simulink library "SUB_ECU_L4_MABX_HW_Interface_PTC_166"  (R2018a)
settings: Solver=VariableStepAuto  StartTime=0.0  StopTime=10.0  RelTol=1e-3
PostLoadFcn:
  | , if any(exist('dsrtsu_mdlpostloadfcn', 'file') == [2, 3, 6]), try dsrtsu_mdlpostloadfcn('Execute', bdroot); catch fprintf('Error in PostLoadFcn (dsrtsu_mdlpostloadfcn) for model "%s":\n %s\n', bdroot, lasterr); end, end,
undefined symbols (not defined in the file or in its folder): CANR_PROPB_REAX_3_13_CHANNEL_APV, CANR_PROPB_REAX_4_13_CHANNEL_APV, CANR_PROPB_XPR_1_50_CHANNEL_APV, ENUM_CAN_RX_T, ENUM_CAN_TX_T, ENUM_REAX_OPERATION_MODE_T, ENUM_SIGNAL_HEALTH_T, ENUM_XBR_CONTROL_MODE_T, ENUM_XBR_EBI_MODE_T, ENUM_XBR_PASS_THROUGH_ACTIVE_T, ENUM_XBR_PRIORITY_T, ENUM_XPR_INHIBIT_PARK_MANUAL_T, ENUM_XPR_INHIBIT_UNPARK_MANUAL_T, ENUM_XPR_PARK_MANUAL_T, ENUM_XPR_UNPARK_MANUAL_T, PROPB_REAX_1_E4_DES_POS_SIG_SRC_APV, PROPB_REAX_1_E4_DESIRED_OPMODE_APV, PROPB_REAX_1_E4_DESIRED_POSITION_APV, ptc_matlab_lib
libraries: PTC_MBDS_LIB x163, rtican x79, simulink x41, EmE_MBD_Blockset x35, rti1401lib_dio_type4 x8, simulink_need_slupdate x7, $bdroot x5, rti1401lib_adc_type4 x3, rtitasklib x1
(part 25 of 25)

== system SUB_ECU_L4_MABX_HW_Interface_PTC_166/CAN_Out_PTC_166/CAN_TX_5000ms/CAN_TX_RQST_13_E4/TX_CAN5 ==
  Enable : Inport
  RawData : Inport  Port=2
  OperatorEnable : Inport  Port=3
  AND : PTC_MBDS_LIB/MBDS Standard Library/Basic Operations/Logic and Bit Operations/AND  BitwiseMode=off  Inputs=2  UseBitMask=off  BitMask='A7'  OutDataTypeStr=Inherit: Inherit via back propagation  PTC_MBDS_BlockVersion=5.41  PTC_BlockType=PTC_MBDS_AND
      settings: SourceProductName=PACCAR Technical Center MBDS Library
  Data Type Conversion : DataTypeConversion
  Data Type Conversion1 : DataTypeConversion
  Data Type Conversion2 : DataTypeConversion
  Demux : Demux  Outputs=3
  RQST_13_E4 : rtican/RTICAN Transmit (TX)   Reserved1=[]  Reserved2=[]  Reserved3=[]  Reserved4=[]  SfcnMessage=[]  Msg_Struct=[]  BoardTypeNo=[]  BoardNo=[]  ChannelNo=[]  Parameters=[]  DialogFcn=[]  UnitName=[]  Revision=[]  UnitValues=[]  DSProperties=struct('RTI',struct('Version',uint32(5),'BlockType',struct('isSLSource',uint8(1),'isSLSink',uint8(1),'isHWSource',uint8(0),'isHWSink',uint8(0),'isSetup',uint8(0),'isInline',uint8(1),'isNonInline',uint8(0),'isInterrupt',uint8(0),'isChannelwise',uint8(0)),'IOBoardType','RTICAN','UnitType','MESSAGE','Identifier','TX','DialogType','MSVC','BlockSet','RTICAN','SlaveProcessor','CAN'))  RTIBlockInterface=struct('InputPortsWidth',int32([1 1 1]),'InputPortsActive',[1 1 1],'InputPortsName',{{'byte1','byte2','byte3'}},'InputPortsDataType',{{'SS_DOUBLE','SS_DOUBLE','SS_DOUBLE'}},'OutputPortsWidth',int32([1 1 1 1]),'OutputPortsActive',[1 1 1 1],'OutputPortsName',{{['TX status'],['TX time'],['TX delta time'],['TX delay time']}},'DialogFcn','rtican_message_interface_gui','BlockDisplay',{{'','center'}},'IconTransparency','on','InitLevel',3,'BlockName',struct('Token',{{'RQST_13_E4'}}),'SampleTime',{{-1}},'TriggerPort',{{'none'}},'EnablePort',{{'yes'}})  RTIBlockParameters=struct('BoardTypeNo',{{1,'OFF',[]}},'BoardNo',{{3,'ON',[1 16]}},'ChannelNo',{{1,'ON',[1 2]}},'Parameters',{{struct('DataFileSupport',struct('DataFileSelectedMaster',1,'DataFileSelectedLocal',0,'DataFileName','c:\data\svn\truck1571\dbc\mabx_can4_chrisbaltonallstandard.dbc|c:\data\svn\truck1571\dbc\mabx_can4.dbc|','DataFileDate',{{{['11-Nov-2016 14:30:51']}}},'SelectedFile',['<no file selected>']),'Options',struct('StatusSelected',1,'TimeSelected',1,'DeltaTimeSelected',1,'DelayTimeSelected',1,'DelayTimeTXCommandSelected',0,'EncodeSetUnusedBitsToOne',0,'EnableMsgLoopback',0,'TriggerPort',struct('Selected',0,'TriggerType',0),'EnablePortSelected',1,'SignalOnPortnameSelected',1,'UserCoding',struct('Selected',0,'InterfaceFile','UserEncodingFile','FcnName','UserEncodeFcn','InportSelected',0,'InportWidth',1,'OutportSelected',0,'OutportWidth',1),'TerminationMsg',struct('Selected',0,'Byte0_7','0'),'InitialMsg',struct('Selected',0,'Byte0_7','0')),'Message',struct('MsgOnBlocknameSelected',1,'MsgName','RQST_13_E4','MsgIdFormat',1,'MsgId',417993700,'MsgLength',8,'NumSignals',3,'SampleTime',-1,'StartTime',struct('Selected',0,'Value',0),'AutoRepeatTime',struct('Selected',0,'Value',0.1),'Timeout',struct('Selected',0,'Value',0.1),'DelayTime',struct('Selected',0,'Value',0.1),'Signal',struct('SgnName',{'byte1','byte2','byte3'},'SgnStartBit',{0,8,16},'SgnLength',{8,8,8},'SgnType',{0,0,0},'ModeValue',{-1,-1,-1},'DataType',{0,0,0},'ByteLayout',{0,0,0},'Factor',{1,1,1},'Offset',{0,0,0},'SgnComment',{{''},{''},{''}},'SgnUnit',{'','',''},'Min',{0,0,0},'Max',{0,0,0},'SLDataType',{'SS_DOUBLE','SS_DOUBLE','SS_DOUBLE'}),'MsgIdNumFormat',1,'MsgComment',{{['Request message 1']}}),'Version',1.2,'general',struct('isFromLib',0)),'OFF',[]}},'GroupId',{{struct('Group',{{'RTICAN'}},'No',5,'Behavior',{{'NAMECHANGE'}},'BlockType',{{'SINK'}},'NameChangeFlag',0),'OFF',[]}},'SFcnRTICANMessage',{{struct('MsgType','TX','SFcnPortType','Scalar','MsgName','RQST_13_E4','MsgIdFormat','XTD','MsgId',417993700,'MsgLength',8,'NumSignals',3,'SampleTime',-1,'StartTime',struct('Selected','no','Value',0),'AutoRepeatTime',struct('Selected','no','Value',0.1),'Timeout',struct('Selected','no','Value',0.1),'Signal',struct('SgnName',{'byte1','byte2','byte3'},'SgnStartBit',{0,8,16},'SgnLength',{8,8,8},'SgnType',{'standard','standard','standard'},'ModeValue',{-1,-1,-1},'DataType',{['unsigned int'],['unsigned int'],['unsigned int']},'ByteLayout',{['little endian'],['little endian'],['little endian']},'Factor',{1,1,1},'Offset',{0,0,0},'SLDataType',{'SS_DOUBLE','SS_DOUBLE','SS_DOUBLE'}),'StatusSelected','yes','TimeSelected','yes','DeltaTimeSelected','yes','DelayTimeSelected','yes','DelayTimeTXCommandSelected','no','EncodeSetUnusedBitsToOne','no','EnableMsgLoopback','no','TriggerPort',struct('Selected','no','TriggerType',0),'EnablePortSelected','yes','UserCoding',struct('Selected','no','InterfaceFile','UserEncodingFile','FcnName','UserEncodeFcn','InportSelected','no','InportWidth',1,'OutportSelected','no','OutportWidth',1),'TerminationMsg',struct('Selected','no','Byte0','0x00','Byte1','0x00','Byte2','0x00','Byte3','0x00','Byte4','0x00','Byte5','0x00','Byte6','0x00','Byte7','0x00'),'InitialMsg',struct('Selected','no','Byte0','0x00','Byte1','0x00','Byte2','0x00','Byte3','0x00','Byte4','0x00','Byte5','0x00','Byte6','0x00','Byte7','0x00'),'BoardType','DS1','BoardNo',3,'ControllerNo',1),'OFF',[]}},'TLCFileName',{{'rtican_tx_message','OFF',[]}})  RTISFcnParameters=struct('SFcnRTICANMessage','struct','TLCFileName','char')  RTIBlockParaDefault=struct('BoardTypeNo',4302,'BoardNo',1,'ChannelNo',1,'Parameters',struct('DataFileSupport',struct('DataFileSelectedMaster',0,'DataFileSelectedLocal',0,'DataFileName','','DataFileDate','','SelectedFile',['<no file selected>']),'Options',struct('StatusSelected',1,'TimeSelected',1,'DeltaTimeSelected',1,'DelayTimeSelected',1,'DelayTimeTXCommandSelected',0,'EncodeSetUnusedBitsToOne',0,'EnableMsgLoopback',0,'TriggerPort',struct('Selected',0,'TriggerType','rising'),'EnablePortSelected',0,'SignalOnPortnameSelected',1,'UserCoding',struct('Selected',0,'InterfaceFile','UserEncodingFile','FcnName','UserEncodeFcn','InportSelected',0,'InportWidth',1,'OutportSelected',0,'OutportWidth',1),'TerminationMsg',struct('Selected',0,'Byte0_7','0'),'InitialMsg',struct('Selected',0,'Byte0_7','0')),'Message',struct('MsgOnBlocknameSelected',0,'MsgName',['TX Message'],'MsgIdFormat',0,'MsgId',100,'MsgLength',8,'NumSignals',1,'SampleTime',-1,'StartTime',struct('Selected',0,'Value',0),'AutoRepeatTime',struct('Selected',0,'Value',0.1),'Timeout',struct('Selected',0,'Value',0.1),'DelayTime',struct('Selected',0,'Value',0.1),'Signal',struct('SgnName',['TX signal'],'SgnStartBit',0,'SgnLength',8,'SgnType',0,'ModeValue',-1,'DataType',0,'SLDataType','SS_DOUBLE','ByteLayout',0,'Factor',1,'Offset',0,'Min',0,'Max',255,'SgnComment',{{}},'SgnUnit',''),'MsgIdNumFormat',0,'MsgComment',{{''}}),'Version',1.2,'general',struct('isFromLib',1)),'GroupId',struct('Group',{{'RTICAN'}},'No',1,'Behavior',{{'NAMECHANGE'}},'BlockType',{{'SINK'}},'NameChangeFlag',0),'SFcnRTICANMessage',struct('MsgType','TX','MsgName',['TX Message'],'MsgIdFormat','STD','MsgId',100,'MsgLength',2,'NumSignals',1,'SampleTime',-1,'StartTime',struct('Selected','no','Value',0),'AutoRepeatTime',struct('Selected','no','Value',0.1),'Timeout',struct('Selected','no','Value',0.1),'DelayTime',struct('Selected','no','Value',0.1),'Signal',struct('SgnName',['TX signal'],'SgnStartBit',0,'SgnLength',8,'SgnType','standard','ModeValue',-1,'DataType',['unsigned int'],'ByteLayout',['little endian'],'SLDataType','SS_DOUBLE','Factor',1,'Offset',0),'StatusSelected','yes','TimeSelected','yes','DeltaTimeSelected','yes','DelayTimeSelected','yes','EnablePortSelected','no','EnableMsgLoopback','no','DelayTimeTXCommandSelected','no','EncodeSetUnusedBitsToOne','no','UserCoding',struct('Selected','no','InterfaceFile','UserDecodingFile','FcnName','UserDecodeFcn','InportSelected','no','InportWidth',1,'OutportSelected','no','OutportWidth',1),'TerminationMsg',struct('Selected','no','Byte0','0x00','Byte1','0x00','Byte2','0x00','Byte3','0x00','Byte4','0x00','Byte5','0x00','Byte6','0x00','Byte7','0x00'),'InitialMsg',struct('Selected','no','Byte0','0x00','Byte1','0x00','Byte2','0x00','Byte3','0x00','Byte4','0x00','Byte5','0x00','Byte6','0x00','Byte7','0x00'),'TriggerPort',struct('Selected','no','TriggerType','rising'),'BoardType','DS4302','BoardNo',1,'ControllerNo',1,'SFcnPortType','Scalar'),'TLCFileName','rtican_tx_message')
      settings: AttributesFormatString=Group Id: RTICAN5\n  SourceProductName=dSPACE RTI CAN Blockset
  Terminator{,1..3} (4 alike) : Terminator
      settings: InitFcn=|
      | try
      |    MBDS_BlockCallback('Update', gcb);
      | end
  wires:
  Data Type Conversion2/1 -> RQST_13_E4/3
  Data Type Conversion1/1 -> RQST_13_E4/2
  Data Type Conversion/1 -> RQST_13_E4/1
  AND/1 -> RQST_13_E4/Enable
  OperatorEnable/1 -> AND/2
  Demux/3 -> Data Type Conversion2/1
  Demux/2 -> Data Type Conversion1/1
  Demux/1 -> Data Type Conversion/1
  RQST_13_E4/1 -> Terminator/1
  RQST_13_E4/3 -> Terminator2/1
  Enable/1 -> AND/1
  RQST_13_E4/4 -> Terminator3/1
  RQST_13_E4/2 -> Terminator1/1
  RawData/1 -> Demux/1

== system SUB_ECU_L4_MABX_HW_Interface_PTC_166/CAN_Out_PTC_166/CAN_TX_VariableRate/CAN_TX_Std_SystemTime_01/TX_CAN6 ==
  Enable : Inport
  Data : Inport  Port=2
  AND : PTC_MBDS_LIB/MBDS Standard Library/Basic Operations/Logic and Bit Operations/AND  BitwiseMode=off  Inputs=2  UseBitMask=off  BitMask='A7'  OutDataTypeStr=Inherit: Inherit via back propagation  PTC_MBDS_BlockVersion=5.41  PTC_BlockType=PTC_MBDS_AND
      settings: SourceProductName=PACCAR Technical Center MBDS Library
  Bus Selector : BusSelector  OutputSignals=INPUTS.CAN.SystemTime.RX_status,INPUTS.CAN.SystemTime.SID,INPUTS.CAN.SystemTime.Source,INPUTS.CAN.SystemTime.Date,INPUTS.CAN.SystemTime.Time
  Constant : Constant  Value=0
  Constant1 : Constant
  Std_SystemTime_01 : rtican/RTICAN Transmit (TX)   Reserved1=[]  Reserved2=[]  Reserved3=[]  Reserved4=[]  SfcnMessage=[]  Msg_Struct=[]  BoardTypeNo=[]  BoardNo=[]  ChannelNo=[]  Parameters=[]  DialogFcn=[]  UnitName=[]  Revision=[]  UnitValues=[]  DSProperties=struct('RTI',struct('Version',uint32(5),'BlockType',struct('isSLSource',uint8(1),'isSLSink',uint8(1),'isHWSource',uint8(0),'isHWSink',uint8(0),'isSetup',uint8(0),'isInline',uint8(1),'isNonInline',uint8(0),'isInterrupt',uint8(0),'isChannelwise',uint8(0)),'IOBoardType','RTICAN','UnitType','MESSAGE','Identifier','TX','DialogType','MSVC','BlockSet','RTICAN','SlaveProcessor','CAN'))  RTIBlockInterface=struct('InputPortsWidth',int32([1 1 1 1 1 1]),'InputPortsActive',[1 1 1 1 1 1],'InputPortsName',{{'SID','Source','Date','Time',['Delay TX command'],'Loop-back'}},'InputPortsDataType',{{'SS_DOUBLE','SS_DOUBLE','SS_DOUBLE','SS_DOUBLE','SS_DOUBLE','SS_DOUBLE'}},'OutputPortsWidth',int32([1 1 1 1]),'OutputPortsActive',[1 1 1 1],'OutputPortsName',{{['TX status'],['TX time'],['TX delta time'],['TX delay time']}},'DialogFcn','rtican_message_interface_gui','BlockDisplay',{{'','center'}},'IconTransparency','on','InitLevel',3,'BlockName',struct('Token',{{'Std_SystemTime_01'}}),'SampleTime',{{-1}},'TriggerPort',{{'none'}},'EnablePort',{{'yes'}})  RTIBlockParameters="struct('BoardTypeNo',{{1,'OFF',[]}},'BoardNo',{{3,'ON',[1 16]}},'ChannelNo',{{2,'ON',[1 2]}},'Parameters',{{struct('DataFileSupport',struct('DataFileSelectedMaster',1,'DataFileSelectedLocal',1,'DataFileName','c:\\localdata\\chris\\advanced_tech\\adas\\level4_rcp\\truck1571\\dbc\\mabx_can6.dbc|c:\\localdata\\chris\\advanced_tech\\adas\\level4_rcp\\candb\\mabx_can4_chrisbalton.dbc|','DataFileDate',['15-Feb-2018 08:21:11'],'SelectedFile','dbc\\mabx_can6_beta4.dbc','InterfaceFcn','rtican_dbc_file_parser'),'Options',struct('StatusSelected',1,'TimeSelected',1,'DeltaTimeSelected',1,'DelayTimeSelected',1,'DelayTimeTXCommandSelected',1,'EncodeSetUnusedBitsToOne',0,'EnableMsgLoopback',1,'TriggerPort',struct('Selected',0,'TriggerType',0),'EnablePortSelected',1,'SignalOnPortnameSelected',1,'UserCoding',struct('Selected',0,'InterfaceFile','UserEncodingFile','FcnName','UserEncodeFcn','InportSelected',0,'InportWidth',1,'OutportSelected',0,'OutportWidth',1),'TerminationMsg',struct('Selected',0,'Byte0_7','0'),'InitialMsg',struct('Selected',0,'Byte0_7','0')),'Message',struct('MsgOnBlocknameSelected',1,'MsgName','Std_SystemTime_01','MsgIdFormat',0,'MsgId',5,'MsgLength',8,'NumSignals',4,'SampleTime',-1,'StartTime',struct('Selected',0,'Value',0),'AutoRepeatTime',struct('Selected',0,'Value',0.1),'Timeout',struct('Selected',0,'Value',0.1),'DelayTime',struct('Selected',0,'Value',0.1),'Signal',struct('SgnName',{'SID','Source','Date','Time'},'SgnStartBit',{0,8,16,32},'SgnLength',{8,4,16,32},'ByteLayout',{0,0,0,0},'Factor',{1,1,1,0.0001},'Offset',{0,0,0,0},'SgnComment',{['An upward counting number used to tie related information together between different PGNs.For example,SID would be used to tie together COG,SOG and RAIM values to a given Pos.255=no valid Pos fix to tie it to.Range 0 to 250 for valid Pos fixes.'],['0x0 = GPS, ' char(10) '0x1 =GLONASS, ' char(10) '0x2 = WWV or equivalent Radio Station Time Sync, ' char(10) '0x3 = Local Cesium clock, ' char(10) '0x4 = Local Rubidium clock, ' char(10) '0x5 = Local Crystal clock, ' char(10) '0x6 - 0xE = reserved, ' char(10) '0xF = Null'],['Days since January 1, 1970,   Date is relative to UTC Time.'],['24 hour clock, 0 =  midnight,  time is in UTC']},'SgnUnit',{'','','day','sec'},'Min',{0,0,0,0},'Max',{252,15,65532,86401},'SgnType',{0,0,0,0},'SLDataType',{'SS_DOUBLE','SS_DOUBLE','SS_DOUBLE','SS_DOUBLE'},'DataType',{0,0,0,0},'ModeValue',{-1,-1,-1,-1}),'MsgIdNumFormat',0,'MsgComment',{{['The purpose of this PGN is twofold:' char(10) '' char(10) '- To provide a regular transmission of UTC time and date' char(10) '- To provide synchronism for measurement data']}}),'Version',1.2,'general',struct('isFromLib',0)),'OFF',[]}},'GroupId',{{struct('Group',{{'RTICAN'}},'No',6,'Behavior',{{'NAMECHANGE'}},'BlockType',{{'SINK'}},'NameChangeFlag',0),'OFF',[]}},'SFcnRTICANMessage',{{struct('MsgType','TX','SFcnPortType','Scalar','MsgName','Std_SystemTime_01','MsgIdFormat','STD','MsgId',5,'MsgLength',8,'NumSignals',4,'SampleTime',-1,'StartTime',struct('Selected','no','Value',0),'AutoRepeatTime',struct('Selected','no','Value',0.1),'Timeout',struct('Selected','no','Value',0.1),'Signal',struct('SgnName',{'SID','Source','Date','Time'},'SgnStartBit',{0,8,16,32},'SgnLength',{8,4,16,32},'ByteLayout',{['little endian'],['little endian'],['little endian'],['little endian']},'Factor',{1,1,1,0.0001},'Offset',{0,0,0,0},'SgnType',{'standard','standard','standard','standard'},'SLDataType',{'SS_DOUBLE','SS_DOUBLE','SS_DOUBLE','SS_DOUBLE'},'DataType',{['unsigned int'],['unsigned int'],['unsigned int'],['unsigned int']},'ModeValue',{-1,-1,-1,-1}),'StatusSelected','yes','TimeSelected','yes','DeltaTimeSelected','yes','DelayTimeSelected','yes','DelayTimeTXCommandSelected','yes','EncodeSetUnusedBitsToOne','no','EnableMsgLoopback','yes','TriggerPort',struct('Selected','no','TriggerType',0),'EnablePortSelected','yes','UserCoding',struct('Selected','no','InterfaceFile','UserEncodingFile','FcnName','UserEncodeFcn','InportSelected','no','InportWidth',1,'OutportSelected','no','OutportWidth',1),'TerminationMsg',struct('Selected','no','Byte0','0x00','Byte1','0x00','Byte2','0x00','Byte3','0x00','Byte4','0x00','Byte5','0x00','Byte6','0x00','Byte7','0x00'),'InitialMsg',struct('Selected','no','Byte0','0x00','Byte1','0x00','Byte2','0x00','Byte3','0x00','Byte4','0x00','Byte5','0x00','Byte6','0x00','Byte7','0x00'),'BoardType','DS1','BoardNo',3,'ControllerNo',2),'OFF',[]}},'TLCFileName',{{'rtican_tx_message','OFF',[]}})"  RTISFcnParameters=struct('SFcnRTICANMessage','struct','TLCFileName','char')  RTIBlockParaDefault=struct('BoardTypeNo',4302,'BoardNo',1,'ChannelNo',1,'Parameters',struct('DataFileSupport',struct('DataFileSelectedMaster',0,'DataFileSelectedLocal',0,'DataFileName','','DataFileDate','','SelectedFile',['<no file selected>']),'Options',struct('StatusSelected',1,'TimeSelected',1,'DeltaTimeSelected',1,'DelayTimeSelected',1,'DelayTimeTXCommandSelected',0,'EncodeSetUnusedBitsToOne',0,'EnableMsgLoopback',0,'TriggerPort',struct('Selected',0,'TriggerType','rising'),'EnablePortSelected',0,'SignalOnPortnameSelected',1,'UserCoding',struct('Selected',0,'InterfaceFile','UserEncodingFile','FcnName','UserEncodeFcn','InportSelected',0,'InportWidth',1,'OutportSelected',0,'OutportWidth',1),'TerminationMsg',struct('Selected',0,'Byte0_7','0'),'InitialMsg',struct('Selected',0,'Byte0_7','0')),'Message',struct('MsgOnBlocknameSelected',0,'MsgName',['TX Message'],'MsgIdFormat',0,'MsgId',100,'MsgLength',8,'NumSignals',1,'SampleTime',-1,'StartTime',struct('Selected',0,'Value',0),'AutoRepeatTime',struct('Selected',0,'Value',0.1),'Timeout',struct('Selected',0,'Value',0.1),'DelayTime',struct('Selected',0,'Value',0.1),'Signal',struct('SgnName',['TX signal'],'SgnStartBit',0,'SgnLength',8,'SgnType',0,'ModeValue',-1,'DataType',0,'SLDataType','SS_DOUBLE','ByteLayout',0,'Factor',1,'Offset',0,'Min',0,'Max',255,'SgnComment',{{}},'SgnUnit',''),'MsgIdNumFormat',0,'MsgComment',{{''}}),'Version',1.2,'general',struct('isFromLib',1)),'GroupId',struct('Group',{{'RTICAN'}},'No',1,'Behavior',{{'NAMECHANGE'}},'BlockType',{{'SINK'}},'NameChangeFlag',0),'SFcnRTICANMessage',struct('MsgType','TX','MsgName',['TX Message'],'MsgIdFormat','STD','MsgId',100,'MsgLength',2,'NumSignals',1,'SampleTime',-1,'StartTime',struct('Selected','no','Value',0),'AutoRepeatTime',struct('Selected','no','Value',0.1),'Timeout',struct('Selected','no','Value',0.1),'DelayTime',struct('Selected','no','Value',0.1),'Signal',struct('SgnName',['TX signal'],'SgnStartBit',0,'SgnLength',8,'SgnType','standard','ModeValue',-1,'DataType',['unsigned int'],'ByteLayout',['little endian'],'SLDataType','SS_DOUBLE','Factor',1,'Offset',0),'StatusSelected','yes','TimeSelected','yes','DeltaTimeSelected','yes','DelayTimeSelected','yes','EnablePortSelected','no','EnableMsgLoopback','no','DelayTimeTXCommandSelected','no','EncodeSetUnusedBitsToOne','no','UserCoding',struct('Selected','no','InterfaceFile','UserDecodingFile','FcnName','UserDecodeFcn','InportSelected','no','InportWidth',1,'OutportSelected','no','OutportWidth',1),'TerminationMsg',struct('Selected','no','Byte0','0x00','Byte1','0x00','Byte2','0x00','Byte3','0x00','Byte4','0x00','Byte5','0x00','Byte6','0x00','Byte7','0x00'),'InitialMsg',struct('Selected','no','Byte0','0x00','Byte1','0x00','Byte2','0x00','Byte3','0x00','Byte4','0x00','Byte5','0x00','Byte6','0x00','Byte7','0x00'),'TriggerPort',struct('Selected','no','TriggerType','rising'),'BoardType','DS4302','BoardNo',1,'ControllerNo',1,'SFcnPortType','Scalar'),'TLCFileName','rtican_tx_message')
      settings: AttributesFormatString=Group Id: RTICAN6\n  SourceProductName=dSPACE RTI CAN Blockset
  Terminator{,1..3} (4 alike) : Terminator
      settings: InitFcn=|
      | try
      |    MBDS_BlockCallback('Update', gcb);
      | end
  wires:
  Bus Selector/5 -> Std_SystemTime_01/4  "<Time>"
  Bus Selector/4 -> Std_SystemTime_01/3  "<Date>"
  Bus Selector/3 -> Std_SystemTime_01/2  "<Source>"
  Bus Selector/2 -> Std_SystemTime_01/1  "<SID>"
  Data/1 -> Bus Selector/1
  Constant1/1 -> Std_SystemTime_01/6
  Constant/1 -> Std_SystemTime_01/5
  Std_SystemTime_01/2 -> Terminator1/1
  Std_SystemTime_01/4 -> Terminator3/1
  Std_SystemTime_01/3 -> Terminator2/1
  Std_SystemTime_01/1 -> Terminator/1
  Enable/1 -> AND/1
  Bus Selector/1 -> AND/2  "<RX_status>"
  AND/1 -> Std_SystemTime_01/Enable

== system SUB_ECU_L4_MABX_HW_Interface_PTC_166/CAN_Truck166/CAN_RX_EC1_00/CAN_RX_EC1_00/Decode ==
  Inport : Inport
  timeStamp : Inport  Port=2
  Enable : EnablePort
  Selector : Selector  InputPortWidth=39  IndexOptions=Index vector (dialog)  Indices=1:39  OutputSizes=1
  Subtract : Sum  Inputs=+-  OutDataTypeStr=single  SaturateOnIntegerOverflow=on  InputSameDT=on
      settings: AttributesFormatString=Saturate: %<SaturateOnIntegerOverflow>
  Unit_Delay : UnitDelay  SampleTime=-1
      settings: AttributesFormatString=Init = %<InitialCondition>
  RawData : Outport
  RX_time : Outport  Port=2
  RX_delta_time : Outport  Port=3
  wires:
  Selector/1 -> RawData/1
  Inport/1 -> Selector/1
  Subtract/1 -> RX_delta_time/1
  Unit_Delay/1 -> Subtract/2
  timeStamp/1 -> RX_time/1, Subtract/1, Unit_Delay/1

== system SUB_ECU_L4_MABX_HW_Interface_PTC_166/CAN_Truck166/CAN_RX_VI_00/CAN_RX_VI_00/Decode ==
  Inport : Inport
  timeStamp : Inport  Port=2
  Enable : EnablePort
  Selector : Selector  InputPortWidth=17  IndexOptions=Index vector (dialog)  Indices=1:17  OutputSizes=1
  Subtract : Sum  Inputs=+-  OutDataTypeStr=single  SaturateOnIntegerOverflow=on  InputSameDT=on
      settings: AttributesFormatString=Saturate: %<SaturateOnIntegerOverflow>
  Unit_Delay : UnitDelay  SampleTime=-1
      settings: AttributesFormatString=Init = %<InitialCondition>
  RawData : Outport
  RX_time : Outport  Port=2
  RX_delta_time : Outport  Port=3
  wires:
  timeStamp/1 -> Unit_Delay/1, Subtract/1, RX_time/1
  Unit_Delay/1 -> Subtract/2
  Subtract/1 -> RX_delta_time/1
  Inport/1 -> Selector/1
  Selector/1 -> RawData/1

== system SUB_ECU_L4_MABX_HW_Interface_PTC_166/DIGITAL/PWM pedal input management/Diagnose pedal input signals/Leaky_bucket ==
  Signal_valid_range_max : Inport
  Signal_valid_range_min : Inport  Port=2
  Count_Max : Inport  Port=3
  Count_Min : Inport  Port=4
  Input_signal : Inport  Port=5
  Check Dynamic Range1 : simulink/Model Verification/Check  Dynamic Range  Description=min < u < max  enabled=on  stopWhenAssertionFail=off  export=on  icon=graphic
      settings: SourceProductName=Simulink  SourceProductBaseCode=SL
  Decrement Real World3 : simulink/Additional Math & Discrete/Additional Math: Increment - Decrement/Decrement Real World
      settings: SourceProductName=Simulink  SourceProductBaseCode=SL
  Dynamic_saturation3 : EmE_MBD_Blockset/Discontinuities/Dynamic_saturation
      settings: SourceProductName=PACCAR EmE MBD Blockset
  If_Then_Else3 : EmE_MBD_Blockset/Signal Routing/If_Then_Else
      settings: SourceProductName=PACCAR EmE MBD Blockset
  Increment Real World3 : simulink/Additional Math & Discrete/Additional Math: Increment - Decrement/Increment Real World
      settings: SourceProductName=Simulink  SourceProductBaseCode=SL
  Relational Operator8 : RelationalOperator  Operator=<=  OutDataTypeStr=boolean  RndMeth=Nearest
  Relational Operator9 : RelationalOperator  Operator=~=  OutDataTypeStr=boolean  RndMeth=Nearest
  Unit Delay External IC3 : simulink_need_slupdate/Unit Delay External IC  tsamp=-1
      settings: SourceProductName=Simulink  SourceProductBaseCode=SL
  Fault_Count : Outport
  F_Fault_Soft : Outport  Port=2
  F_Fault_Hard : Outport  Port=3
  wires:
  If_Then_Else3/1 -> Dynamic_saturation3/2
  Signal_valid_range_min/1 -> Check Dynamic Range1/2
  Check Dynamic Range1/1 -> If_Then_Else3/1  "f_signal_valid"
  Signal_valid_range_max/1 -> Check Dynamic Range1/1
  Relational Operator8/1 -> F_Fault_Hard/1  "F_Fault_Hard"
  Count_Max/1 -> Dynamic_saturation3/1, Relational Operator8/1
  Unit Delay External IC3/1 -> Decrement Real World3/1, Increment Real World3/1
  Input_signal/1 -> Check Dynamic Range1/3
  Relational Operator9/1 -> F_Fault_Soft/1  "F_Fault_Soft"
  Increment Real World3/1 -> If_Then_Else3/3
  Decrement Real World3/1 -> If_Then_Else3/2
  Dynamic_saturation3/1 -> Relational Operator8/2, Fault_Count/1, Unit Delay External IC3/1, Relational Operator9/1  "Fault_Count"
  Count_Min/1 -> Dynamic_saturation3/3, Relational Operator9/2, Unit Delay External IC3/2

== system SUB_ECU_L4_MABX_HW_Interface_PTC_166/DIGITAL/PWM pedal input management/Diagnose pedal input signals/Leaky_bucket1 ==
  Signal_valid_range_max : Inport
  Signal_valid_range_min : Inport  Port=2
  Count_Max : Inport  Port=3
  Count_Min : Inport  Port=4
  Input_signal : Inport  Port=5
  Check Dynamic Range1 : simulink/Model Verification/Check  Dynamic Range  Description=min < u < max  enabled=on  stopWhenAssertionFail=off  export=on  icon=graphic
      settings: SourceProductName=Simulink  SourceProductBaseCode=SL
  Decrement Real World3 : simulink/Additional Math & Discrete/Additional Math: Increment - Decrement/Decrement Real World
      settings: SourceProductName=Simulink  SourceProductBaseCode=SL
  Dynamic_saturation3 : EmE_MBD_Blockset/Discontinuities/Dynamic_saturation
      settings: SourceProductName=PACCAR EmE MBD Blockset
  If_Then_Else3 : EmE_MBD_Blockset/Signal Routing/If_Then_Else
      settings: SourceProductName=PACCAR EmE MBD Blockset
  Increment Real World3 : simulink/Additional Math & Discrete/Additional Math: Increment - Decrement/Increment Real World
      settings: SourceProductName=Simulink  SourceProductBaseCode=SL
  Relational Operator8 : RelationalOperator  Operator=<=  OutDataTypeStr=boolean  RndMeth=Nearest
  Relational Operator9 : RelationalOperator  Operator=~=  OutDataTypeStr=boolean  RndMeth=Nearest
  Unit Delay External IC3 : simulink_need_slupdate/Unit Delay External IC  tsamp=-1
      settings: SourceProductName=Simulink  SourceProductBaseCode=SL
  Fault_Count : Outport
  F_Fault_Soft : Outport  Port=2
  F_Fault_Hard : Outport  Port=3
  wires:
  Count_Min/1 -> Unit Delay External IC3/2, Relational Operator9/2, Dynamic_saturation3/3
  Dynamic_saturation3/1 -> Relational Operator9/1, Unit Delay External IC3/1, Fault_Count/1, Relational Operator8/2  "Fault_Count"
  Decrement Real World3/1 -> If_Then_Else3/2
  Increment Real World3/1 -> If_Then_Else3/3
  Relational Operator9/1 -> F_Fault_Soft/1  "F_Fault_Soft"
  Input_signal/1 -> Check Dynamic Range1/3
  Unit Delay External IC3/1 -> Increment Real World3/1, Decrement Real World3/1
  Count_Max/1 -> Relational Operator8/1, Dynamic_saturation3/1
  Relational Operator8/1 -> F_Fault_Hard/1  "F_Fault_Hard"
  Signal_valid_range_max/1 -> Check Dynamic Range1/1
  Check Dynamic Range1/1 -> If_Then_Else3/1  "f_signal_valid"
  Signal_valid_range_min/1 -> Check Dynamic Range1/2
  If_Then_Else3/1 -> Dynamic_saturation3/2

== system SUB_ECU_L4_MABX_HW_Interface_PTC_166/DIGITAL/PWM pedal input management/Diagnose pedal input signals/Leaky_bucket2 ==
  Signal_valid_range_max : Inport
  Signal_valid_range_min : Inport  Port=2
  Count_Max : Inport  Port=3
  Count_Min : Inport  Port=4
  Input_signal : Inport  Port=5
  Check Dynamic Range1 : simulink/Model Verification/Check  Dynamic Range  Description=min < u < max  enabled=on  stopWhenAssertionFail=off  export=on  icon=graphic
      settings: SourceProductName=Simulink  SourceProductBaseCode=SL
  Decrement Real World3 : simulink/Additional Math & Discrete/Additional Math: Increment - Decrement/Decrement Real World
      settings: SourceProductName=Simulink  SourceProductBaseCode=SL
  Dynamic_saturation3 : EmE_MBD_Blockset/Discontinuities/Dynamic_saturation
      settings: SourceProductName=PACCAR EmE MBD Blockset
  If_Then_Else3 : EmE_MBD_Blockset/Signal Routing/If_Then_Else
      settings: SourceProductName=PACCAR EmE MBD Blockset
  Increment Real World3 : simulink/Additional Math & Discrete/Additional Math: Increment - Decrement/Increment Real World
      settings: SourceProductName=Simulink  SourceProductBaseCode=SL
  Relational Operator8 : RelationalOperator  Operator=<=  OutDataTypeStr=boolean  RndMeth=Nearest
  Relational Operator9 : RelationalOperator  Operator=~=  OutDataTypeStr=boolean  RndMeth=Nearest
  Unit Delay External IC3 : simulink_need_slupdate/Unit Delay External IC  tsamp=-1
      settings: SourceProductName=Simulink  SourceProductBaseCode=SL
  Fault_Count : Outport
  F_Fault_Soft : Outport  Port=2
  F_Fault_Hard : Outport  Port=3
  wires:
  Count_Min/1 -> Unit Delay External IC3/2, Relational Operator9/2, Dynamic_saturation3/3
  Dynamic_saturation3/1 -> Relational Operator9/1, Unit Delay External IC3/1, Fault_Count/1, Relational Operator8/2  "Fault_Count"
  Decrement Real World3/1 -> If_Then_Else3/2
  Increment Real World3/1 -> If_Then_Else3/3
  Relational Operator9/1 -> F_Fault_Soft/1  "F_Fault_Soft"
  Input_signal/1 -> Check Dynamic Range1/3
  Unit Delay External IC3/1 -> Increment Real World3/1, Decrement Real World3/1
  Count_Max/1 -> Relational Operator8/1, Dynamic_saturation3/1
  Relational Operator8/1 -> F_Fault_Hard/1  "F_Fault_Hard"
  Signal_valid_range_max/1 -> Check Dynamic Range1/1
  Check Dynamic Range1/1 -> If_Then_Else3/1  "f_signal_valid"
  Signal_valid_range_min/1 -> Check Dynamic Range1/2
  If_Then_Else3/1 -> Dynamic_saturation3/2

== system SUB_ECU_L4_MABX_HW_Interface_PTC_166/DIGITAL/PWM pedal input management/Diagnose pedal input signals/Leaky_bucket3 ==
  Signal_valid_range_max : Inport
  Signal_valid_range_min : Inport  Port=2
  Count_Max : Inport  Port=3
  Count_Min : Inport  Port=4
  Input_signal : Inport  Port=5
  Check Dynamic Range1 : simulink/Model Verification/Check  Dynamic Range  Description=min < u < max  enabled=on  stopWhenAssertionFail=off  export=on  icon=graphic
      settings: SourceProductName=Simulink  SourceProductBaseCode=SL
  Decrement Real World3 : simulink/Additional Math & Discrete/Additional Math: Increment - Decrement/Decrement Real World
      settings: SourceProductName=Simulink  SourceProductBaseCode=SL
  Dynamic_saturation3 : EmE_MBD_Blockset/Discontinuities/Dynamic_saturation
      settings: SourceProductName=PACCAR EmE MBD Blockset
  If_Then_Else3 : EmE_MBD_Blockset/Signal Routing/If_Then_Else
      settings: SourceProductName=PACCAR EmE MBD Blockset
  Increment Real World3 : simulink/Additional Math & Discrete/Additional Math: Increment - Decrement/Increment Real World
      settings: SourceProductName=Simulink  SourceProductBaseCode=SL
  Relational Operator8 : RelationalOperator  Operator=<=  OutDataTypeStr=boolean  RndMeth=Nearest
  Relational Operator9 : RelationalOperator  Operator=~=  OutDataTypeStr=boolean  RndMeth=Nearest
  Unit Delay External IC3 : simulink_need_slupdate/Unit Delay External IC  tsamp=-1
      settings: SourceProductName=Simulink  SourceProductBaseCode=SL
  Fault_Count : Outport
  F_Fault_Soft : Outport  Port=2
  F_Fault_Hard : Outport  Port=3
  wires:
  If_Then_Else3/1 -> Dynamic_saturation3/2
  Signal_valid_range_min/1 -> Check Dynamic Range1/2
  Check Dynamic Range1/1 -> If_Then_Else3/1  "f_signal_valid"
  Signal_valid_range_max/1 -> Check Dynamic Range1/1
  Relational Operator8/1 -> F_Fault_Hard/1  "F_Fault_Hard"
  Count_Max/1 -> Dynamic_saturation3/1, Relational Operator8/1
  Unit Delay External IC3/1 -> Decrement Real World3/1, Increment Real World3/1
  Input_signal/1 -> Check Dynamic Range1/3
  Relational Operator9/1 -> F_Fault_Soft/1  "F_Fault_Soft"
  Increment Real World3/1 -> If_Then_Else3/3
  Decrement Real World3/1 -> If_Then_Else3/2
  Dynamic_saturation3/1 -> Relational Operator8/2, Fault_Count/1, Unit Delay External IC3/1, Relational Operator9/1  "Fault_Count"
  Count_Min/1 -> Dynamic_saturation3/3, Relational Operator9/2, Unit Delay External IC3/2

== system SUB_ECU_L4_MABX_HW_Interface_PTC_166/DIGITAL/PWM pedal input management/Diagnose pedal input signals/Leaky_bucket4 ==
  Signal_valid_range_max : Inport
  Signal_valid_range_min : Inport  Port=2
  Count_Max : Inport  Port=3
  Count_Min : Inport  Port=4
  Input_signal : Inport  Port=5
  Check Dynamic Range1 : simulink/Model Verification/Check  Dynamic Range  Description=min < u < max  enabled=on  stopWhenAssertionFail=off  export=on  icon=graphic
      settings: SourceProductName=Simulink  SourceProductBaseCode=SL
  Decrement Real World3 : simulink/Additional Math & Discrete/Additional Math: Increment - Decrement/Decrement Real World
      settings: SourceProductName=Simulink  SourceProductBaseCode=SL
  Dynamic_saturation3 : EmE_MBD_Blockset/Discontinuities/Dynamic_saturation
      settings: SourceProductName=PACCAR EmE MBD Blockset
  If_Then_Else3 : EmE_MBD_Blockset/Signal Routing/If_Then_Else
      settings: SourceProductName=PACCAR EmE MBD Blockset
  Increment Real World3 : simulink/Additional Math & Discrete/Additional Math: Increment - Decrement/Increment Real World
      settings: SourceProductName=Simulink  SourceProductBaseCode=SL
  Relational Operator8 : RelationalOperator  Operator=<=  OutDataTypeStr=boolean  RndMeth=Nearest
  Relational Operator9 : RelationalOperator  Operator=~=  OutDataTypeStr=boolean  RndMeth=Nearest
  Unit Delay External IC3 : simulink_need_slupdate/Unit Delay External IC  tsamp=-1
      settings: SourceProductName=Simulink  SourceProductBaseCode=SL
  Fault_Count : Outport
  F_Fault_Soft : Outport  Port=2
  F_Fault_Hard : Outport  Port=3
  wires:
  If_Then_Else3/1 -> Dynamic_saturation3/2
  Signal_valid_range_min/1 -> Check Dynamic Range1/2
  Check Dynamic Range1/1 -> If_Then_Else3/1  "f_signal_valid"
  Signal_valid_range_max/1 -> Check Dynamic Range1/1
  Relational Operator8/1 -> F_Fault_Hard/1  "F_Fault_Hard"
  Count_Max/1 -> Dynamic_saturation3/1, Relational Operator8/1
  Unit Delay External IC3/1 -> Decrement Real World3/1, Increment Real World3/1
  Input_signal/1 -> Check Dynamic Range1/3
  Relational Operator9/1 -> F_Fault_Soft/1  "F_Fault_Soft"
  Increment Real World3/1 -> If_Then_Else3/3
  Decrement Real World3/1 -> If_Then_Else3/2
  Dynamic_saturation3/1 -> Relational Operator8/2, Fault_Count/1, Unit Delay External IC3/1, Relational Operator9/1  "Fault_Count"
  Count_Min/1 -> Dynamic_saturation3/3, Relational Operator9/2, Unit Delay External IC3/2

== system SUB_ECU_L4_MABX_HW_Interface_PTC_166/CAN_Out_PTC_166/CAN_TX_10ms/Encode_PROPB_REAX_1/PropB_REAX_1_E4_CommandFromExternalController/ALL_CTRL_DISABLED ==
  Enable : EnablePort
      settings: AttributesFormatString=States when enabling: %<StatesWhenEnabling>
  Constant : Constant  Value=typecast(uint32(hex2dec('FFFFFFFF')), 'int32')
  Out1 : Outport  InitialOutput=0
      settings: AttributesFormatString=Output when disabled: %<OutputWhenDisabled>
  wires:
  Constant/1 -> Out1/1

== system SUB_ECU_L4_MABX_HW_Interface_PTC_166/CAN_Out_PTC_166/CAN_TX_10ms/Encode_PROPB_REAX_1/PropB_REAX_1_E4_CommandFromExternalController/DEFAULT_TRQ_CTRL_MODE ==
  Enable : EnablePort
      settings: AttributesFormatString=States when enabling: %<StatesWhenEnabling>
  Constant : Constant  Value=typecast(uint32(hex2dec('FFFFFFFF')), 'int32')
  Out1 : Outport  InitialOutput=0
      settings: AttributesFormatString=Output when disabled: %<OutputWhenDisabled>
  wires:
  Constant/1 -> Out1/1

== system SUB_ECU_L4_MABX_HW_Interface_PTC_166/CAN_Out_PTC_166/CAN_TX_10ms/Encode_PROPB_REAX_1/PropB_REAX_1_E4_CommandFromExternalController/Desired_Steering_Angle ==
  DesiredSteeringAngle : Inport
  OperatorEnable : Inport  Port=2
  Constant1 : Constant  Value=PROPB_REAX_1_E4_DES_POS_SIG_SRC_APV
  Constant7 : Constant  Value=PROPB_REAX_1_E4_DESIRED_POSITION_APV
  Multiport_Switch : MultiPortSwitch  DataPortOrder=Specify indices  DataPortIndices={ENUM_STEERING_POS_SIGNAL_SOURCE_T.SW_EMULATION, ENUM_STEERING_POS_SIGNAL_SOURCE_T.ESTIMATION}  DataPortForDefault=Additional data port  SaturateOnIntegerOverflow=on  InputSameDT=on
      settings: AttributesFormatString=Zero-based indexing: %<zeroidx>
  Switch : Switch  Criteria=u2 ~= 0
  zero : Constant  Value=0
  Out1 : Outport
  wires:
  zero/1 -> Switch/3
  Switch/1 -> Out1/1
  OperatorEnable/1 -> Switch/2
  Multiport_Switch/1 -> Switch/1
  DesiredSteeringAngle/1 -> Multiport_Switch/3
  Constant7/1 -> Multiport_Switch/2, Multiport_Switch/4
  Constant1/1 -> Multiport_Switch/1

== system SUB_ECU_L4_MABX_HW_Interface_PTC_166/CAN_Out_PTC_166/CAN_TX_10ms/Encode_PROPB_REAX_1/PropB_REAX_1_E4_CommandFromExternalController/EXT_TRQ_CTRL_MODE_A ==
  Enable : EnablePort
      settings: AttributesFormatString=States when enabling: %<StatesWhenEnabling>
  Constant : Constant  Value=typecast(uint32(hex2dec('FFFFFFFF')), 'int32')
  Out1 : Outport  InitialOutput=0
      settings: AttributesFormatString=Output when disabled: %<OutputWhenDisabled>
  wires:
  Constant/1 -> Out1/1

== system SUB_ECU_L4_MABX_HW_Interface_PTC_166/CAN_Out_PTC_166/CAN_TX_10ms/Encode_PROPB_REAX_1/PropB_REAX_1_E4_CommandFromExternalController/EXT_TRQ_CTRL_MODE_B ==
  Enable : EnablePort
      settings: AttributesFormatString=States when enabling: %<StatesWhenEnabling>
  Constant : Constant  Value=typecast(uint32(hex2dec('FFFFFFFF')), 'int32')
  Out1 : Outport  InitialOutput=0
      settings: AttributesFormatString=Output when disabled: %<OutputWhenDisabled>
  wires:
  Constant/1 -> Out1/1

== system SUB_ECU_L4_MABX_HW_Interface_PTC_166/CAN_Out_PTC_166/CAN_TX_10ms/Encode_PROPB_REAX_1/PropB_REAX_1_E4_CommandFromExternalController/EXT_TRQ_CTRL_MODE_C ==
  Enable : EnablePort
      settings: AttributesFormatString=States when enabling: %<StatesWhenEnabling>
  Constant : Constant  Value=typecast(uint32(hex2dec('FFFFFFFF')), 'int32')
  Out1 : Outport  InitialOutput=0
      settings: AttributesFormatString=Output when disabled: %<OutputWhenDisabled>
  wires:
  Constant/1 -> Out1/1

== system SUB_ECU_L4_MABX_HW_Interface_PTC_166/CAN_Out_PTC_166/CAN_TX_10ms/Encode_PROPB_REAX_1/PropB_REAX_1_E4_CommandFromExternalController/POSITION_CONTROL_MODE ==
  In1 : Inport
  Enable : EnablePort
      settings: AttributesFormatString=States when enabling: %<StatesWhenEnabling>
  Constant : Constant  Value=8192/360
  Data Type Conversion : DataTypeConversion  OutDataTypeStr=int32  SaturateOnIntegerOverflow=on
  Product : Product  Inputs=**  OutDataTypeStr=Inherit: Inherit via back propagation  SaturateOnIntegerOverflow=on  InputSameDT=on
      settings: AttributesFormatString=Saturate: %<SaturateOnIntegerOverflow>
  Out1 : Outport  InitialOutput=0
      settings: AttributesFormatString=Output when disabled: %<OutputWhenDisabled>
  wires:
  Data Type Conversion/1 -> Out1/1
  Product/1 -> Data Type Conversion/1
  Constant/1 -> Product/2
  In1/1 -> Product/1

== matlab function SUB_ECU_L4_MABX_HW_Interface_PTC_166/CAN_Truck166/CAN_RX_EC1_00/CAN_RX_EC1_00/serialize_tpdt ==
  data: RX_status output boolean; data_packet_previous input uint8; Data output uint8; TotalNumberOfPackets input uint8; SequenceNumber input uint8; byte1 input uint8; byte2 input uint8; byte3 input uint8; byte4 input uint8; byte5 input uint8; byte6 input uint8; byte7 input uint8
function [RX_status, Data] = serialize_tpdt(data_packet_previous, ...
    TotalNumberOfPackets, ...
    SequenceNumber, byte1, byte2, byte3, byte4, byte5, byte6, byte7)
%#codegen

if SequenceNumber > 1
    Data = data_packet_previous;
else
    Data = uint8(255) * ones(39, 1, 'uint8');
end
starting_index = 7*SequenceNumber - 6;
Data(starting_index : starting_index + 6) = [byte1; byte2; byte3; byte4; byte5; byte6; byte7];
RX_status = (SequenceNumber == TotalNumberOfPackets);

end

== stateflow chart SUB_ECU_L4_MABX_HW_Interface_PTC_166/CAN_Out_PTC_166/CAN_TX_BAM/Chart ==
  state Init
    en:State= uint8(0);
    en:enTPCM=logical(0);
    en:enTPDT=logical(0);
    en:TPCM_ts_Prev=TPCM_ts;
    en:TPDT_ts_Prev=TPDT_ts;
    en:TPDT_count=uint8(0);
  state StartMsg
    en:State= uint8(1);
    en:TPDT_count=uint8(1);
  state SendTPCM
    en:State=uint8(2);
    en:enTPCM=logical(1);
  state InterframeDelay
    en:State=uint8(3);
    en:enTPCM=logical(0);
    en:TPCM_ts_Prev=TPCM_ts;
  state SendTPDT
    en:State=uint8(4);
    en:enTPDT=logical(1);
  state InterframeDelay1
    en:State= uint8(5);
    en:enTPDT=logical(0);
    en:TPDT_ts_Prev=TPDT_ts;
  state CheckPacketCount
    en:State=uint8(6);
    en:TPDT_count=TPDT_count+uint8(1);
  state WaitForNextPeriod
    en:State=uint8(7);
  (default) -> Init
  Init -> StartMsg
  WaitForNextPeriod -> StartMsg : after(1.85,sec)
  StartMsg -> SendTPCM
  SendTPCM -> InterframeDelay : after(.010,sec)
  InterframeDelay -> SendTPDT : after(0.05, sec)
  CheckPacketCount -> SendTPDT [order 1] : [TPDT_count<=TPDT_total]
  SendTPDT -> InterframeDelay1 : after(0.01,sec)
  InterframeDelay1 -> CheckPacketCount : after(0.05,sec)
  CheckPacketCount -> WaitForNextPeriod [order 2]
  data: State output uint8; enTPDT output boolean; enTPCM output boolean; TPCM_ts input; TPDT_ts input; TPCM_ts_Prev output; TPDT_ts_Prev output; TPDT_count output uint8; TPDT_total input uint8

== stateflow chart SUB_ECU_L4_MABX_HW_Interface_PTC_166/DIGITAL/RationalityCheck/Chart ==
  state init
    en:DiagPassed=logical(0);
  state SwitchOff
  state SwitchOn
  state DiagPassed
    en:DiagPassed=logical(1);
  (default) -> init
  init -> SwitchOn [order 2] : [Input==1]
  init -> SwitchOff [order 1] : [Input==0]
  SwitchOff -> DiagPassed : [Input==1]
  SwitchOn -> SwitchOff : [Input==0]
  data: Input input boolean; DiagPassed output boolean

== stateflow chart SUB_ECU_L4_MABX_HW_Interface_PTC_166/DIGITAL/PWM pedal input management/Diagnose pedal input signals/Health State Machine PWM Sensor 1 ==
  state NO_FAILURE
    en: Pedal_1_pwm_health_state = ENUM_SIGNAL_HEALTH_T.FAULT_INACTIVE;
  state FAILURE_DETECTED
    state PENDING
      en: Pedal_1_pwm_health_state = ENUM_SIGNAL_HEALTH_T.FAULT_PENDING;
    state ERROR
      en: Pedal_1_pwm_health_state = ENUM_SIGNAL_HEALTH_T.FAULT_ACTIVE;
    (default) -> PENDING
    PENDING -> ERROR [order 2] : [F_Pedal_1_pwm_fault_active]
    ERROR -> PENDING : [~F_Pedal_1_pwm_fault_active]
  (default) -> NO_FAILURE
  NO_FAILURE -> FAILURE_DETECTED : [F_Pedal_1_pwm_fault_pending || ...
      | F_Pedal_1_pwm_fault_active]
  PENDING -> NO_FAILURE [order 1] : [~F_Pedal_1_pwm_fault_pending && ...
      | ~F_Pedal_1_pwm_fault_active]
  data: F_Pedal_1_pwm_fault_pending input; F_Pedal_1_pwm_fault_active input; Pedal_1_pwm_health_state output Enum: ENUM_SIGNAL_HEALTH_T

== stateflow chart SUB_ECU_L4_MABX_HW_Interface_PTC_166/DIGITAL/PWM pedal input management/Diagnose pedal input signals/Health State Machine PWM Sensor 2 ==
  state NO_FAILURE
    en: Pedal_2_pwm_health_state = ENUM_SIGNAL_HEALTH_T.FAULT_INACTIVE;
  state FAILURE_DETECTED
    state PENDING
      en: Pedal_2_pwm_health_state = ENUM_SIGNAL_HEALTH_T.FAULT_PENDING;
    state ERROR
      en: Pedal_2_pwm_health_state = ENUM_SIGNAL_HEALTH_T.FAULT_ACTIVE;
    (default) -> PENDING
    PENDING -> ERROR [order 2] : [F_Pedal_2_pwm_fault_active]
    ERROR -> PENDING : [~F_Pedal_2_pwm_fault_active]
  (default) -> NO_FAILURE
  NO_FAILURE -> FAILURE_DETECTED : [F_Pedal_2_pwm_fault_pending || ...
      | F_Pedal_2_pwm_fault_active]
  PENDING -> NO_FAILURE [order 1] : [~F_Pedal_2_pwm_fault_pending && ...
      | ~F_Pedal_2_pwm_fault_active]
  data: F_Pedal_2_pwm_fault_pending input; F_Pedal_2_pwm_fault_active input; Pedal_2_pwm_health_state output

== matlab function SUB_ECU_L4_MABX_HW_Interface_PTC_166/CAN_Truck166/CAN_RX_VI_00/CAN_RX_VI_00/serialize_tpdt ==
  data: RX_status output boolean; data_packet_previous input uint8; Data output uint8; TotalNumberOfPackets input uint8; SequenceNumber input uint8; byte1 input uint8; byte2 input uint8; byte3 input uint8; byte4 input uint8; byte5 input uint8; byte6 input uint8; byte7 input uint8
function [RX_status, Data] = serialize_tpdt(data_packet_previous, ...
    TotalNumberOfPackets, ...
    SequenceNumber, byte1, byte2, byte3, byte4, byte5, byte6, byte7)
%#codegen

if SequenceNumber > 1
    Data = data_packet_previous;
else
    Data = uint8(255) * ones(17, 1, 'uint8');
end
starting_index = 7*SequenceNumber - 6;
Data(starting_index : starting_index + 6) = [byte1; byte2; byte3; byte4; byte5; byte6; byte7];
RX_status = (SequenceNumber == TotalNumberOfPackets);

end
